simulink model "CLLLC_Plant_vLoad_V2"  (R2022a)
settings: Solver=FixedStepDiscrete  StartTime=0.0  StopTime=0.5  FixedStep=Step_Rate  RelTol=1e-3
model workspace (MAT data in the model file):
  CVI_INit = 0
  Fsw : Simulink.Signal (value not decoded)
  L_Lim = 0.6
  fnerr : Simulink.Signal (value not decoded)
  fsw : Simulink.Signal (value not decoded)
  swit : Simulink.Signal (value not decoded)
  tsw : Simulink.Signal (value not decoded)
values from neighbouring files (symbols this model uses):
  a0_cv_F = 0.01392699    [CLLLC_Plant_Parameters_vLoad_V2.m]
  a1_cv_F = -0.0060730    (= -0.006073)    [CLLLC_Plant_Parameters_vLoad_V2.m]
  a2_cv_F = 0.0    (= 0)    [CLLLC_Plant_Parameters_vLoad_V2.m]
  b1_cv_F = -1    [CLLLC_Plant_Parameters_vLoad_V2.m]
  b2_cv_F = 0.0    (= 0)    [CLLLC_Plant_Parameters_vLoad_V2.m]
  Cmd_Ref_Ctrl = round(Cmd_Ref * KVpri / VADC * ADCFS)    [CLLLC_Plant_Parameters_vLoad_V2.m]
  Control_Step_Rate = 50e-6    (= 5e-05)    [CLLLC_Plant_Parameters_vLoad_V2.m]
  Freq_Sw = 55.1e3    (= 55100)    [CLLLC_Plant_Parameters_vLoad_V2.m]
  KIout = 20e-3    (= 0.02)    [CLLLC_Plant_Parameters_vLoad_V2.m]
  KVpri = 0.0036102    [CLLLC_Plant_Parameters_vLoad_V2.m]
  KVsec = 0.00569815    [CLLLC_Plant_Parameters_vLoad_V2.m]
  Lm1 = Ln*LrP1    (= 8e-05)    [CLLLC_Plant_Parameters_vLoad_V2.m]
  n = 20.0/9.0    (= 2.22222222222)    [CLLLC_Plant_Parameters_vLoad_V2.m]
  R_series = 3    [CLLLC_Plant_Parameters_vLoad_V2.m]
  Reverse = 1    [CLLLC_Plant_Parameters_vLoad_V2.m]
  Step_Rate = 1e-7    (= 1e-07)    [CLLLC_Plant_Parameters_vLoad_V2.m]
  transformerCoupling = 0.999    [CLLLC_Plant_Parameters_vLoad_V2.m]
  Ts_Sw = floor(Fclk/Freq_Sw)    [CLLLC_Plant_Parameters_vLoad_V2.m]
libraries: fl_lib x36, nesl_utility x25, ee_lib x15, simulink x7, spsFirstOrderFilterLib x5, slpidlib x3, simulink_extras x3, eeGeneralControl x1
(part 3 of 3)

== system CLLLC_Plant_vLoad_V2/Loop Selection/Open Loop 1 ==
  note: 0 - SR Disable
      | 1 - SR Enable
  Constant : Constant  Value=0
  Mode Selection : Subsystem  Variant=on
  PWM_freq : Outport
  SR_En : Outport  Port=2
  wires:
  Constant/1 -> SR_En/1
  Mode Selection/1(PWM_Freq) -> PWM_freq/1

== system CLLLC_Plant_vLoad_V2/Loop Selection/Closed Loop/Mode Selection ==
  note: 1) Add Subsystem or Model blocks as valid variant choices.
      | 2) You cannot connect blocks at this level. At simulation, connectivity is automatically
      | determined, based on the active variant and port name matching.
  CC Mode : Subsystem  VariantControl=Charger_Mode == 0
  CV Mode Forward : Subsystem  VariantControl=Charger_Mode == 1
  CV Mode Reverse : Subsystem  VariantControl=Charger_Mode == 2
  PWM_Freq : Outport

== system CLLLC_Plant_vLoad_V2/Loop Selection/Closed Loop1/Mode Selection ==
  note: 1) Add Subsystem or Model blocks as valid variant choices.
      | 2) You cannot connect blocks at this level. At simulation, connectivity is automatically
      | determined, based on the active variant and port name matching.
  CC Mode : Subsystem  VariantControl=Charger_Mode == 0
  CV Mode Forward : Subsystem  VariantControl=Charger_Mode == 1
  CV Mode Reverse : Subsystem  VariantControl=Charger_Mode == 2
  PWM_freq : Outport

== system CLLLC_Plant_vLoad_V2/Loop Selection/Open Loop 1/Mode Selection ==
  note: 1) Add Subsystem or Model blocks as valid variant choices.
      | 2) You cannot connect blocks at this level. At simulation, connectivity is automatically
      | determined, based on the active variant and port name matching.
  CC Mode : Subsystem  VariantControl=Charger_Mode == 0
  CV Mode : Subsystem  VariantControl=Charger_Mode == 1
  PWM_Freq : Outport

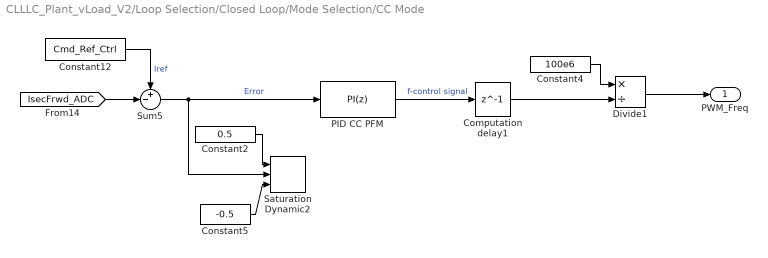
== system CLLLC_Plant_vLoad_V2/Loop Selection/Closed Loop/Mode Selection/CC Mode ==
  Computation delay1 : Delay  DelayLength=1  InitialCondition=200
  Constant12 : Constant  Value=Cmd_Ref_Ctrl
  Constant2 : Constant  Value=0.5
  Constant4 : Constant  Value=100e6
  Constant5 : Constant  Value=-0.5
  Divide1 : Product  Inputs=*/
  PID CC PFM : slpidlib/PID Controller  Controller=PI  Form=Parallel  TimeDomain=Discrete-time  UseExternalTs=off  SampleTime=Control_Step_Rate  IntegratorMethod=Forward Euler  FilterMethod=Forward Euler  ControllerParametersSource=internal  P=0.0661065319076132  I=416.251558932139  UseKiTs=off  D=-0.0462494978274742  N=100  UseFilter=off  TunerSelectOption=Transfer Function Based (PID Tuner App)  InitialConditionSource=internal  InitialConditionForIntegrator=200  InitialConditionForFilter=0  DifferentiatorICPrevScaledInput=0  ExternalReset=none  TrackingMode=off  Kt=1  LimitOutput=on  SatLimitsSource=internal  UpperSaturationLimit=750  LowerSaturationLimit=200  LinearizeAsGain=on  AntiWindupMode=back-calculation  Kb=1  POutMin=[]  POutMax=[]  IOutMin=[]  IOutMax=[]  DOutMin=[]  DOutMax=[]  NOutMin=[]  NOutMax=[]  SumOutMin=[]  SumOutMax=[]  SaturationOutMin=[]  SaturationOutMax=[]  PParamMin=[]  PParamMax=[]  IParamMin=[]  IParamMax=[]  DParamMin=[]  DParamMax=[]  NParamMin=[]  NParamMax=[]  KbParamMin=[]  KbParamMax=[]  KtParamMin=[]  KtParamMax=[]  KbOutMin=[]  KbOutMax=[]  KtOutMin=[]  KtOutMax=[]  IntegratorOutMin=[]  IntegratorOutMax=[]  FilterOutMin=[]  FilterOutMax=[]  SumI1OutMin=[]  SumI1OutMax=[]  SumI2OutMin=[]  SumI2OutMax=[]  SumI3OutMin=[]  SumI3OutMax=[]  SumI4OutMin=[]  SumI4OutMax=[]  SumDOutMin=[]  SumDOutMax=[]  DifferentiatorOutMin=[]  DifferentiatorOutMax=[]  FilterDiffOutCoefMin=[]  FilterDiffOutCoefMax=[]  ReciprocalOutMin=[]  ReciprocalOutMax=[]  SumDenOutMin=[]  SumDenOutMax=[]  SumNumOutMin=[]  SumNumOutMax=[]  DivideOutMin=[]  DivideOutMax=[]  UdiffTsProdOutMin=[]  UdiffTsProdOutMax=[]  NTsProdOutMin=[]  NTsProdOutMax=[]  UintegralTsProdOutMin=[]  UintegralTsProdOutMax=[]  UngainTsProdOutMin=[]  UngainTsProdOutMax=[]  IntegratorContinuousStateAttributes=''  IntegratorStateMustResolveToSignalObject=off  IntegratorRTWStateStorageClass=Auto  FilterContinuousStateAttributes=''  FilterStateMustResolveToSignalObject=off  FilterRTWStateStorageClass=Auto  ParallelPVariant=InternalParameters  IdealPVariant=Disabled  IVariant=InternalParameters  DVariant=Disabled  IntegratorVariant=Discrete  SatVariant=Enabled  AWVariant=BackCalculation  PCopyVariant=Disabled  TRVariant=Disabled  FdbkBlocksVariant=Forward  IdealPFdbkVariant=Disabled  SatFdbkVariant=Disabled  DerivativeFilterVariant=Disabled  NVariant=Disabled  NCopyVariant=Disabled_SignalSpec  FilterICVariant=Disabled  IntegratorICVariant=InternalICs  ExternalResetVariant=Disabled  TRSumVariant=Passthrough  SumFdbkVariant=Disabled  SumVariant=Sum_PI  TsampFilterVariant=InternalTs  TsampNgainVariant=Passthrough  TsampIntegralVariant=Passthrough  ExternalSaturationOutDataTypeStr=Inherit: Same as second input  aMode=0
  Saturation Dynamic2 : simulink/Discontinuities/Saturation Dynamic  OutMin=[]  OutMax=[]  OutDataTypeStr=Inherit: Same as second input  OutDataType=fixdt(1, 16)  OutScaling=2^-10  DoSatur=off
  Sum5 : Sum  Inputs=+-|
  PWM_Freq : Outport
  wires:
  PID CC PFM/1 -> Computation delay1/1  "f-control signal"
  Constant2/1 -> Saturation Dynamic2/1
  Sum5/1 -> Saturation Dynamic2/2, PID CC PFM/1  "Error"
  Constant5/1 -> Saturation Dynamic2/3
  [IsecFrwd_ADC] -> Sum5/2
  Constant12/1 -> Sum5/1  "Iref"
  Constant4/1 -> Divide1/1
  Computation delay1/1 -> Divide1/2
  Divide1/1 -> PWM_Freq/1

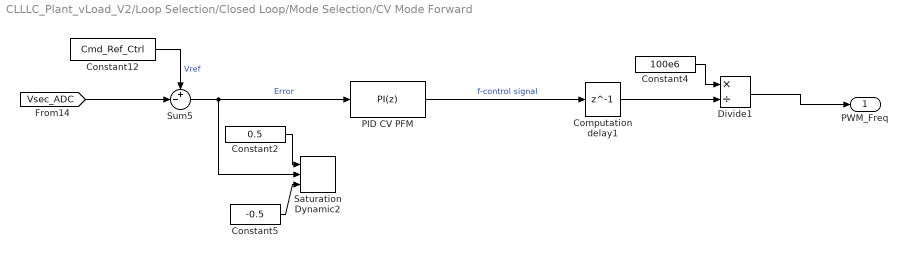
== system CLLLC_Plant_vLoad_V2/Loop Selection/Closed Loop/Mode Selection/CV Mode Forward ==
  Computation delay1 : Delay  DelayLength=1  InitialCondition=200
  Constant12 : Constant  Value=Cmd_Ref_Ctrl
  Constant2 : Constant  Value=0.5
  Constant4 : Constant  Value=100e6
  Constant5 : Constant  Value=-0.5
  Divide1 : Product  Inputs=*/
  PID CV PFM : slpidlib/PID Controller  Controller=PI  Form=Parallel  TimeDomain=Discrete-time  UseExternalTs=off  SampleTime=Control_Step_Rate  IntegratorMethod=Forward Euler  FilterMethod=Forward Euler  ControllerParametersSource=internal  P=0.068496  I=349.9686  UseKiTs=off  D=-0.0462494978274742  N=100  UseFilter=off  TunerSelectOption=Transfer Function Based (PID Tuner App)  InitialConditionSource=internal  InitialConditionForIntegrator=200  InitialConditionForFilter=0  DifferentiatorICPrevScaledInput=0  ExternalReset=none  TrackingMode=off  Kt=1  LimitOutput=on  SatLimitsSource=internal  UpperSaturationLimit=750  LowerSaturationLimit=200  LinearizeAsGain=on  AntiWindupMode=back-calculation  Kb=1  POutMin=[]  POutMax=[]  IOutMin=[]  IOutMax=[]  DOutMin=[]  DOutMax=[]  NOutMin=[]  NOutMax=[]  SumOutMin=[]  SumOutMax=[]  SaturationOutMin=[]  SaturationOutMax=[]  PParamMin=[]  PParamMax=[]  IParamMin=[]  IParamMax=[]  DParamMin=[]  DParamMax=[]  NParamMin=[]  NParamMax=[]  KbParamMin=[]  KbParamMax=[]  KtParamMin=[]  KtParamMax=[]  KbOutMin=[]  KbOutMax=[]  KtOutMin=[]  KtOutMax=[]  IntegratorOutMin=[]  IntegratorOutMax=[]  FilterOutMin=[]  FilterOutMax=[]  SumI1OutMin=[]  SumI1OutMax=[]  SumI2OutMin=[]  SumI2OutMax=[]  SumI3OutMin=[]  SumI3OutMax=[]  SumI4OutMin=[]  SumI4OutMax=[]  SumDOutMin=[]  SumDOutMax=[]  DifferentiatorOutMin=[]  DifferentiatorOutMax=[]  FilterDiffOutCoefMin=[]  FilterDiffOutCoefMax=[]  ReciprocalOutMin=[]  ReciprocalOutMax=[]  SumDenOutMin=[]  SumDenOutMax=[]  SumNumOutMin=[]  SumNumOutMax=[]  DivideOutMin=[]  DivideOutMax=[]  UdiffTsProdOutMin=[]  UdiffTsProdOutMax=[]  NTsProdOutMin=[]  NTsProdOutMax=[]  UintegralTsProdOutMin=[]  UintegralTsProdOutMax=[]  UngainTsProdOutMin=[]  UngainTsProdOutMax=[]  IntegratorContinuousStateAttributes=''  IntegratorStateMustResolveToSignalObject=off  IntegratorRTWStateStorageClass=Auto  FilterContinuousStateAttributes=''  FilterStateMustResolveToSignalObject=off  FilterRTWStateStorageClass=Auto  ParallelPVariant=InternalParameters  IdealPVariant=Disabled  IVariant=InternalParameters  DVariant=Disabled  IntegratorVariant=Discrete  SatVariant=Enabled  AWVariant=BackCalculation  PCopyVariant=Disabled  TRVariant=Disabled  FdbkBlocksVariant=Forward  IdealPFdbkVariant=Disabled  SatFdbkVariant=Disabled  DerivativeFilterVariant=Disabled  NVariant=Disabled  NCopyVariant=Disabled_SignalSpec  FilterICVariant=Disabled  IntegratorICVariant=InternalICs  ExternalResetVariant=Disabled  TRSumVariant=Passthrough  SumFdbkVariant=Disabled  SumVariant=Sum_PI  TsampFilterVariant=InternalTs  TsampNgainVariant=Passthrough  TsampIntegralVariant=Passthrough  ExternalSaturationOutDataTypeStr=Inherit: Same as second input  aMode=0
  Saturation Dynamic2 : simulink/Discontinuities/Saturation Dynamic  OutMin=[]  OutMax=[]  OutDataTypeStr=Inherit: Same as second input  OutDataType=fixdt(1, 16)  OutScaling=2^-10  DoSatur=off
  Sum5 : Sum  Inputs=+-|
  PWM_Freq : Outport
  wires:
  Constant2/1 -> Saturation Dynamic2/1
  Sum5/1 -> Saturation Dynamic2/2, PID CV PFM/1  "Error"
  Constant5/1 -> Saturation Dynamic2/3
  PID CV PFM/1 -> Computation delay1/1  "f-control signal"
  Constant12/1 -> Sum5/1  "Vref"
  Constant4/1 -> Divide1/1
  Divide1/1 -> PWM_Freq/1
  [Vsec_ADC] -> Sum5/2
  Computation delay1/1 -> Divide1/2

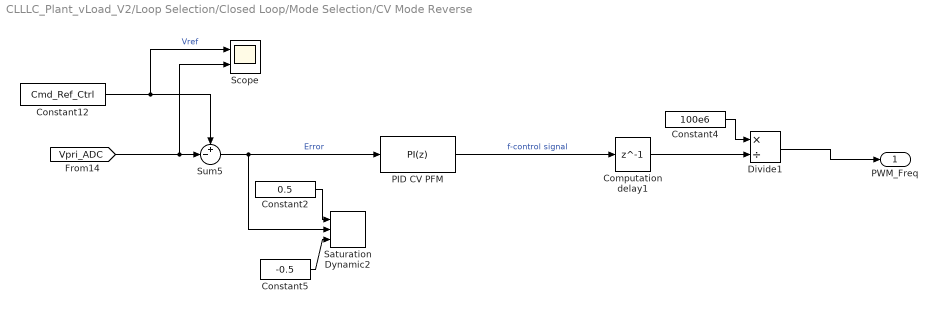
== system CLLLC_Plant_vLoad_V2/Loop Selection/Closed Loop/Mode Selection/CV Mode Reverse ==
  Computation delay1 : Delay  DelayLength=1  InitialCondition=200
  Constant12 : Constant  Value=Cmd_Ref_Ctrl
  Constant2 : Constant  Value=0.5
  Constant4 : Constant  Value=100e6
  Constant5 : Constant  Value=-0.5
  Divide1 : Product  Inputs=*/
  PID CV PFM : slpidlib/PID Controller  Controller=PI  Form=Parallel  TimeDomain=Discrete-time  UseExternalTs=off  SampleTime=Control_Step_Rate  IntegratorMethod=Forward Euler  FilterMethod=Forward Euler  ControllerParametersSource=internal  P=0.170506780572651  I=9.31712886047831  UseKiTs=off  D=-0.0462494978274742  N=100  UseFilter=off  TunerSelectOption=Transfer Function Based (PID Tuner App)  InitialConditionSource=internal  InitialConditionForIntegrator=361  InitialConditionForFilter=0  DifferentiatorICPrevScaledInput=0  ExternalReset=none  TrackingMode=off  Kt=1  LimitOutput=on  SatLimitsSource=internal  UpperSaturationLimit=750  LowerSaturationLimit=200  LinearizeAsGain=on  AntiWindupMode=back-calculation  Kb=1  POutMin=[]  POutMax=[]  IOutMin=[]  IOutMax=[]  DOutMin=[]  DOutMax=[]  NOutMin=[]  NOutMax=[]  SumOutMin=[]  SumOutMax=[]  SaturationOutMin=[]  SaturationOutMax=[]  PParamMin=[]  PParamMax=[]  IParamMin=[]  IParamMax=[]  DParamMin=[]  DParamMax=[]  NParamMin=[]  NParamMax=[]  KbParamMin=[]  KbParamMax=[]  KtParamMin=[]  KtParamMax=[]  KbOutMin=[]  KbOutMax=[]  KtOutMin=[]  KtOutMax=[]  IntegratorOutMin=[]  IntegratorOutMax=[]  FilterOutMin=[]  FilterOutMax=[]  SumI1OutMin=[]  SumI1OutMax=[]  SumI2OutMin=[]  SumI2OutMax=[]  SumI3OutMin=[]  SumI3OutMax=[]  SumI4OutMin=[]  SumI4OutMax=[]  SumDOutMin=[]  SumDOutMax=[]  DifferentiatorOutMin=[]  DifferentiatorOutMax=[]  FilterDiffOutCoefMin=[]  FilterDiffOutCoefMax=[]  ReciprocalOutMin=[]  ReciprocalOutMax=[]  SumDenOutMin=[]  SumDenOutMax=[]  SumNumOutMin=[]  SumNumOutMax=[]  DivideOutMin=[]  DivideOutMax=[]  UdiffTsProdOutMin=[]  UdiffTsProdOutMax=[]  NTsProdOutMin=[]  NTsProdOutMax=[]  UintegralTsProdOutMin=[]  UintegralTsProdOutMax=[]  UngainTsProdOutMin=[]  UngainTsProdOutMax=[]  IntegratorContinuousStateAttributes=''  IntegratorStateMustResolveToSignalObject=off  IntegratorRTWStateStorageClass=Auto  FilterContinuousStateAttributes=''  FilterStateMustResolveToSignalObject=off  FilterRTWStateStorageClass=Auto  ParallelPVariant=InternalParameters  IdealPVariant=Disabled  IVariant=InternalParameters  DVariant=Disabled  IntegratorVariant=Discrete  SatVariant=Enabled  AWVariant=BackCalculation  PCopyVariant=Disabled  TRVariant=Disabled  FdbkBlocksVariant=Forward  IdealPFdbkVariant=Disabled  SatFdbkVariant=Disabled  DerivativeFilterVariant=Disabled  NVariant=Disabled  NCopyVariant=Disabled_SignalSpec  FilterICVariant=Disabled  IntegratorICVariant=InternalICs  ExternalResetVariant=Disabled  TRSumVariant=Passthrough  SumFdbkVariant=Disabled  SumVariant=Sum_PI  TsampFilterVariant=InternalTs  TsampNgainVariant=Passthrough  TsampIntegralVariant=Passthrough  ExternalSaturationOutDataTypeStr=Inherit: Same as second input  aMode=0
  Saturation Dynamic2 : simulink/Discontinuities/Saturation Dynamic  OutMin=[]  OutMax=[]  OutDataTypeStr=Inherit: Same as second input  OutDataType=fixdt(1, 16)  OutScaling=2^-10  DoSatur=off
  Scope : Scope  NumInputPorts=2
  Sum5 : Sum  Inputs=+-|
  PWM_Freq : Outport
  wires:
  Constant2/1 -> Saturation Dynamic2/1
  Sum5/1 -> Saturation Dynamic2/2, PID CV PFM/1  "Error"
  Constant5/1 -> Saturation Dynamic2/3
  PID CV PFM/1 -> Computation delay1/1  "f-control signal"
  Constant12/1 -> Scope/1, Sum5/1  "Vref"
  Constant4/1 -> Divide1/1
  Divide1/1 -> PWM_Freq/1
  [Vpri_ADC] -> Scope/2, Sum5/2
  Computation delay1/1 -> Divide1/2

== system CLLLC_Plant_vLoad_V2/Loop Selection/Closed Loop1/Mode Selection/CC Mode ==
  Constant12 : Constant  Value=Cmd_Ref_Ctrl
  Subsystem : Subsystem
  PWM_freq : Outport
  wires:
  [IsecFrwd_ADC] -> Subsystem/2(In2)
  [Control_step_timer] -> Subsystem/Trigger
  Subsystem/1(PWM_freq) -> PWM_freq/1
  Constant12/1 -> Subsystem/1(Iref)  "Iref"

== system CLLLC_Plant_vLoad_V2/Loop Selection/Closed Loop1/Mode Selection/CV Mode Forward ==
  Constant12 : Constant  Value=Cmd_Ref_Ctrl
  Subsystem : Subsystem
  PWM_freq : Outport
  wires:
  Constant12/1 -> Subsystem/1(Vref)  "Vref"
  [Vsec_ADC] -> Subsystem/2(In2)
  Subsystem/1(Out1) -> PWM_freq/1
  [Control_step_timer] -> Subsystem/Trigger

== system CLLLC_Plant_vLoad_V2/Loop Selection/Closed Loop1/Mode Selection/CV Mode Reverse ==
  Constant12 : Constant  Value=Cmd_Ref_Ctrl
  Subsystem : Subsystem
  PWM_freq : Outport
  wires:
  Constant12/1 -> Subsystem/1(Vref)  "Vref"
  [Vpri_ADC] -> Subsystem/2(In2)
  Subsystem/1(Out1) -> PWM_freq/1
  [Control_step_timer] -> Subsystem/Trigger

== system CLLLC_Plant_vLoad_V2/Loop Selection/Open Loop 1/Mode Selection/CC Mode ==
  Constant4 : Constant  Value=100e6
  Constant5 : Constant  Value=Ts_Sw
  Divide1 : Product  Inputs=*/
  PWM_Freq : Outport
  wires:
  Constant5/1 -> Divide1/2  "f-control signal"
  Constant4/1 -> Divide1/1
  Divide1/1 -> PWM_Freq/1

== system CLLLC_Plant_vLoad_V2/Loop Selection/Open Loop 1/Mode Selection/CV Mode ==
  note: f-control signal
  Constant4 : Constant  Value=100e6
  Constant5 : Constant  Value=Ts_Sw
  Divide1 : Product  Inputs=*/
  PWM_Freq : Outport
  wires:
  Constant5/1 -> Divide1/2
  Constant4/1 -> Divide1/1
  Divide1/1 -> PWM_Freq/1

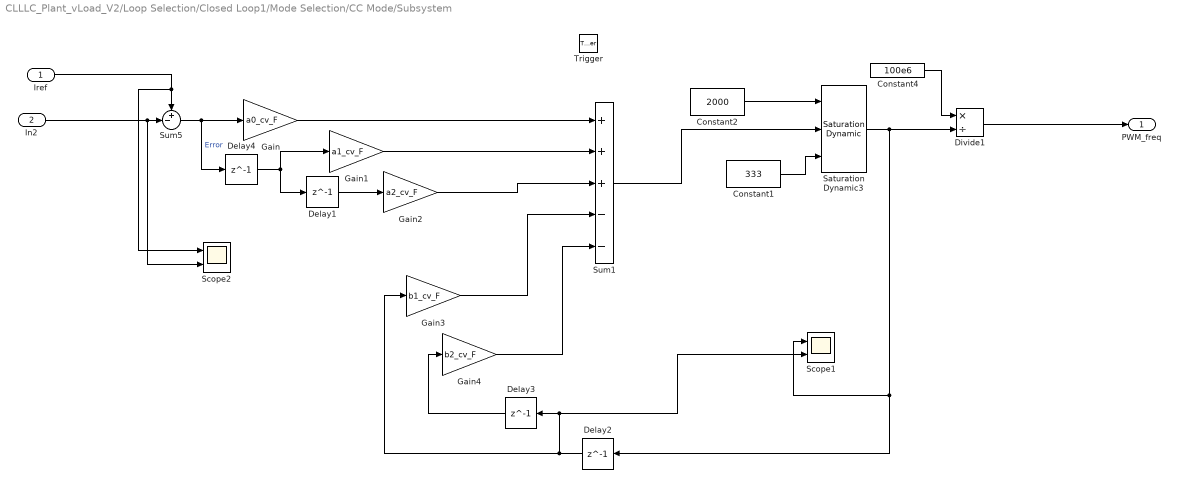
== system CLLLC_Plant_vLoad_V2/Loop Selection/Closed Loop1/Mode Selection/CC Mode/Subsystem ==
  Iref : Inport
  In2 : Inport  Port=2
  Trigger : TriggerPort  VariantControl=Variant  PortDimensions=1
  Constant1 : Constant  Value=333  OutDataTypeStr=single
  Constant2 : Constant  Value=2000  OutDataTypeStr=single
  Constant4 : Constant  Value=100e6
  Delay1 : Delay  DelayLength=1  InitialCondition=0
  Delay2 : Delay  DelayLength=1  InitialCondition=125
  Delay3 : Delay  DelayLength=1  InitialCondition=125
  Delay4 : Delay  DelayLength=1  InitialCondition=0
  Divide1 : Product  Inputs=*/
  Gain : Gain  Gain=a0_cv_F
  Gain1 : Gain  Gain=a1_cv_F
  Gain2 : Gain  Gain=a2_cv_F
  Gain3 : Gain  Gain=b1_cv_F
  Gain4 : Gain  Gain=b2_cv_F
  Saturation Dynamic3 : simulink/Discontinuities/Saturation Dynamic  OutMin=[]  OutMax=[]  OutDataTypeStr=Inherit: Same as second input  OutDataType=fixdt(1, 16)  OutScaling=2^-10  DoSatur=off
  Scope1 : Scope  NumInputPorts=2
  Scope2 : Scope  NumInputPorts=2
  Sum1 : Sum  Inputs=+++--
  Sum5 : Sum  Inputs=+-|
  PWM_freq : Outport
  wires:
  Saturation Dynamic3/1 -> Delay2/1, Scope1/1, Divide1/2
  Constant1/1 -> Saturation Dynamic3/3
  Sum5/1 -> Gain/1, Delay4/1  "Error"
  Gain3/1 -> Sum1/4
  Constant2/1 -> Saturation Dynamic3/1
  Delay1/1 -> Gain2/1
  Gain1/1 -> Sum1/2
  Delay4/1 -> Delay1/1, Gain1/1
  Sum1/1 -> Saturation Dynamic3/2
  Delay3/1 -> Gain4/1
  Delay2/1 -> Gain3/1, Scope1/2, Delay3/1
  Divide1/1 -> PWM_freq/1
  Gain/1 -> Sum1/1
  Iref/1 -> Sum5/1, Scope2/1
  Gain4/1 -> Sum1/5
  Gain2/1 -> Sum1/3
  Constant4/1 -> Divide1/1
  In2/1 -> Scope2/2, Sum5/2

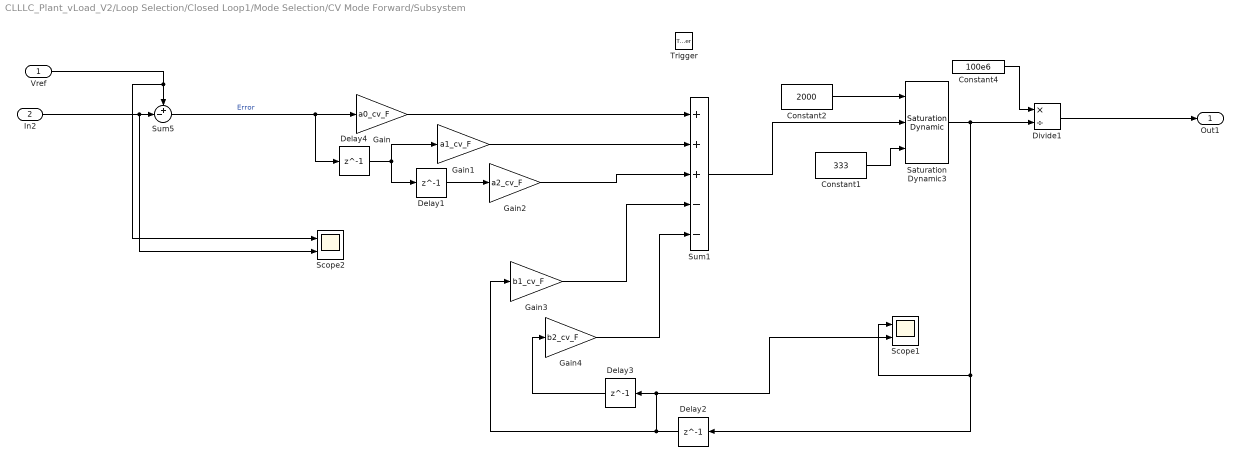
== system CLLLC_Plant_vLoad_V2/Loop Selection/Closed Loop1/Mode Selection/CV Mode Forward/Subsystem ==
  Vref : Inport
  In2 : Inport  Port=2
  Trigger : TriggerPort  VariantControl=Variant  PortDimensions=1
  Constant1 : Constant  Value=333  OutDataTypeStr=single
  Constant2 : Constant  Value=2000  OutDataTypeStr=single
  Constant4 : Constant  Value=100e6
  Delay1 : Delay  DelayLength=1  InitialCondition=0
  Delay2 : Delay  DelayLength=1  InitialCondition=125
  Delay3 : Delay  DelayLength=1  InitialCondition=125
  Delay4 : Delay  DelayLength=1  InitialCondition=0
  Divide1 : Product  Inputs=*/
  Gain : Gain  Gain=a0_cv_F
  Gain1 : Gain  Gain=a1_cv_F
  Gain2 : Gain  Gain=a2_cv_F
  Gain3 : Gain  Gain=b1_cv_F
  Gain4 : Gain  Gain=b2_cv_F
  Saturation Dynamic3 : simulink/Discontinuities/Saturation Dynamic  OutMin=[]  OutMax=[]  OutDataTypeStr=Inherit: Same as second input  OutDataType=fixdt(1, 16)  OutScaling=2^-10  DoSatur=off
  Scope1 : Scope  NumInputPorts=2
  Scope2 : Scope  NumInputPorts=2
  Sum1 : Sum  Inputs=+++--
  Sum5 : Sum  Inputs=+-|
  Out1 : Outport
  wires:
  Saturation Dynamic3/1 -> Delay2/1, Scope1/1, Divide1/2
  Constant1/1 -> Saturation Dynamic3/3
  Sum5/1 -> Gain/1, Delay4/1  "Error"
  Gain3/1 -> Sum1/4
  Constant2/1 -> Saturation Dynamic3/1
  Delay1/1 -> Gain2/1
  Gain1/1 -> Sum1/2
  Delay4/1 -> Delay1/1, Gain1/1
  Sum1/1 -> Saturation Dynamic3/2
  Delay3/1 -> Gain4/1
  Delay2/1 -> Gain3/1, Scope1/2, Delay3/1
  Divide1/1 -> Out1/1
  Gain/1 -> Sum1/1
  Vref/1 -> Sum5/1, Scope2/1
  Gain4/1 -> Sum1/5
  Gain2/1 -> Sum1/3
  Constant4/1 -> Divide1/1
  In2/1 -> Scope2/2, Sum5/2

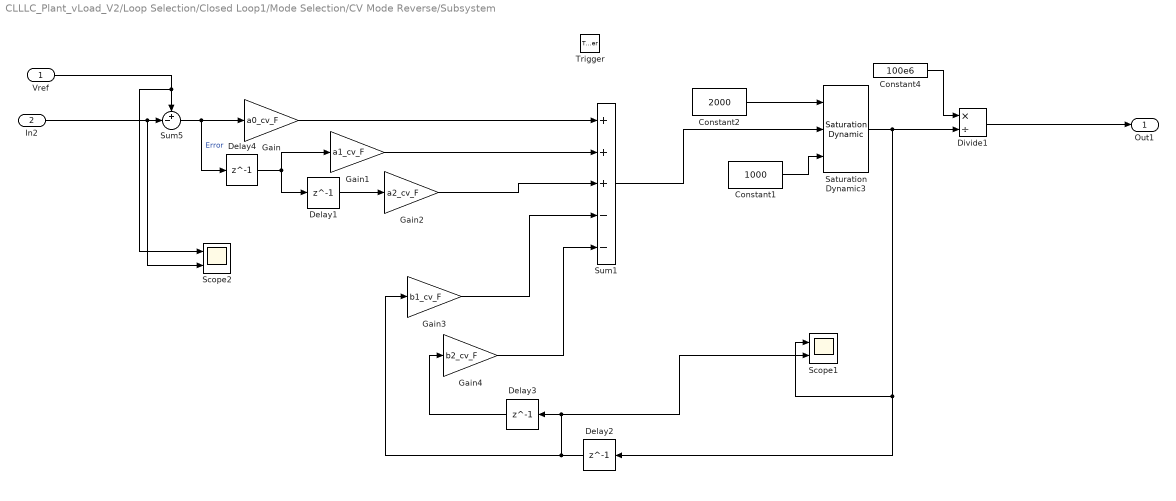
== system CLLLC_Plant_vLoad_V2/Loop Selection/Closed Loop1/Mode Selection/CV Mode Reverse/Subsystem ==
  Vref : Inport
  In2 : Inport  Port=2
  Trigger : TriggerPort  VariantControl=Variant  PortDimensions=1
  Constant1 : Constant  Value=1000  OutDataTypeStr=single
  Constant2 : Constant  Value=2000  OutDataTypeStr=single
  Constant4 : Constant  Value=100e6
  Delay1 : Delay  DelayLength=1  InitialCondition=0
  Delay2 : Delay  DelayLength=1  InitialCondition=346
  Delay3 : Delay  DelayLength=1  InitialCondition=346
  Delay4 : Delay  DelayLength=1  InitialCondition=0
  Divide1 : Product  Inputs=*/
  Gain : Gain  Gain=a0_cv_F
  Gain1 : Gain  Gain=a1_cv_F
  Gain2 : Gain  Gain=a2_cv_F
  Gain3 : Gain  Gain=b1_cv_F
  Gain4 : Gain  Gain=b2_cv_F
  Saturation Dynamic3 : simulink/Discontinuities/Saturation Dynamic  OutMin=[]  OutMax=[]  OutDataTypeStr=Inherit: Same as second input  OutDataType=fixdt(1, 16)  OutScaling=2^-10  DoSatur=off
  Scope1 : Scope  NumInputPorts=2
  Scope2 : Scope  NumInputPorts=2
  Sum1 : Sum  Inputs=+++--
  Sum5 : Sum  Inputs=+-|
  Out1 : Outport
  wires:
  Saturation Dynamic3/1 -> Delay2/1, Scope1/1, Divide1/2
  Constant1/1 -> Saturation Dynamic3/3
  Sum5/1 -> Gain/1, Delay4/1  "Error"
  Gain3/1 -> Sum1/4
  Constant2/1 -> Saturation Dynamic3/1
  Delay1/1 -> Gain2/1
  Gain1/1 -> Sum1/2
  Delay4/1 -> Delay1/1, Gain1/1
  Sum1/1 -> Saturation Dynamic3/2
  Delay3/1 -> Gain4/1
  Delay2/1 -> Gain3/1, Scope1/2, Delay3/1
  Divide1/1 -> Out1/1
  Gain/1 -> Sum1/1
  Vref/1 -> Sum5/1, Scope2/1
  Gain4/1 -> Sum1/5
  Gain2/1 -> Sum1/3
  Constant4/1 -> Divide1/1
  In2/1 -> Scope2/2, Sum5/2

== matlab function CLLLC_Plant_vLoad_V2/Loop Selection/Open Loop/Open Loop Soft Start ==
  settings: updateMethod=DISCRETE
  data: Step_Rate parameter; PWM_Freq output; SR_EN output; Freq_Sw parameter
function [PWM_Freq, SR_EN] = OpenLoopSS(Step_Rate, Freq_Sw)
 
persistent PWM_Freq_Start
if isempty(PWM_Freq_Start) %Init
    PWM_Freq_Start = 200e3;
end
 
persistent PWM_Freq_Curr1
if isempty(PWM_Freq_Curr1) %Init
    PWM_Freq_Curr1 = PWM_Freq_Start;
end
 
persistent SS_Flag1
if isempty(SS_Flag1) %Init
    SS_Flag1 = 0;
end
 
Freq_Step = (PWM_Freq_Start - Freq_Sw) / (0.0001/Step_Rate);
 
if SS_Flag1 == 0
    if PWM_Freq_Curr1 <= Freq_Sw 
        SS_Flag1 = 1;
    else
        PWM_Freq_Curr1 = PWM_Freq_Curr1 - Freq_Step;
    end
else
    PWM_Freq_Curr1 = Freq_Sw;
end
 
PWM_Freq = PWM_Freq_Curr1;
 
if SS_Flag1 == 1 
    SR_EN = 0;
else
    SR_EN = 0;
end
 
end

== matlab function CLLLC_Plant_vLoad_V2/PWM Generator  CLLLC ==
  settings: updateMethod=DISCRETE
  data: PWM_Freq input; SR_En input; Step_Rate parameter; Reverse parameter; PWMPA output; PWMPB output; PWMSA output; PWMSB output; PRD output
function [PWMPA, PWMPB, PWMSA, PWMSB, PRD]   = PWM_Generator(PWM_Freq, SR_En, Step_Rate, Reverse)
 
persistent Period_Act
if isempty(Period_Act) %Init
    Period_Act = 0;
end
 
persistent Period_Count
if isempty(Period_Count) %Init
    Period_Count = 0;
end
 
persistent PWM1A_Stat 
if isempty(PWM1A_Stat) %Init
    PWM1A_Stat = 0;
end
 
persistent PWM1B_Stat 
if isempty(PWM1B_Stat) %Init
    PWM1B_Stat = 0;
end
 
persistent PWM2A_Stat 
if isempty(PWM2A_Stat) %Init
    PWM2A_Stat = 0;
end
 
persistent PWM2B_Stat 
if isempty(PWM2B_Stat) %Init
    PWM2B_Stat = 0;
end
 
persistent PWM1A_H 
if isempty(PWM1A_H) %Init
    PWM1A_H = 0;
end
 
persistent PWM1A_L 
if isempty(PWM1A_L) %Init
    PWM1A_L = 0;
end
 
persistent PWM1B_H 
if isempty(PWM1B_H) %Init
    PWM1B_H = 0;
end
 
persistent PWM1B_L 
if isempty(PWM1B_L) %Init
    PWM1B_L = 0;
end
 
persistent PWM2A_H 
if isempty(PWM2A_H) %Init
    PWM2A_H = 0;
end
 
persistent PWM2A_L 
if isempty(PWM2A_L) %Init
    PWM2A_L = 0;
end
 
persistent PWM2B_H 
if isempty(PWM2B_H) %Init
    PWM2B_H = 0;
end
 
persistent PWM2B_L 
if isempty(PWM2B_L) %Init
    PWM2B_L = 0;
end
 
Pri_Dead_Time = 0.25e-6 / Step_Rate;
Sec_Dead_Time = 0.5e-6 / Step_Rate;
 
Pri_DTime_Half_Count = Pri_Dead_Time / 2;
Sec_DTime_Half_Count = Sec_Dead_Time / 2;
 
if PWM_Freq <= 0
    PWM_Freq = 240000;
end
    
Period_Cmd = (1/PWM_Freq) / Step_Rate;
 
if Period_Count >= Period_Act
    Period_Count = 0;
        
    Period_Act = Period_Cmd;
        
    % Update Duty Count
    Duty_50 = Period_Cmd / 2;
    
    %Base Frequecny PWM With 50% Duty
    PWM1A_H = Pri_DTime_Half_Count;
    PWM1A_L = Duty_50 - Pri_DTime_Half_Count;      % -1 to Avoid Overflow
    
    PWM1B_H = Duty_50 + Pri_DTime_Half_Count;
    PWM1B_L = Period_Cmd - Pri_DTime_Half_Count;
    
    %With Phase Shift
    PWM2A_H = Sec_DTime_Half_Count;
    PWM2A_L = Duty_50 - Sec_DTime_Half_Count;      % -1 to Avoid Overflow
    
    PWM2B_H = Duty_50 + Sec_DTime_Half_Count;
    PWM2B_L = Period_Cmd - Sec_DTime_Half_Count;    
else
     Period_Count = Period_Count + 1; 
end
 
if Period_Count > PWM1A_L 
    PWM1A_Stat = 0;
elseif Period_Count > PWM1A_H       
    PWM1A_Stat = 1;
end
 
if Period_Count > PWM1B_L 
    PWM1B_Stat = 0;
elseif Period_Count > PWM1B_H         
    PWM1B_Stat = 1;
end
 
if Period_Count > PWM2A_L 
    PWM2A_Stat = 0;
elseif Period_Count > PWM2A_H       
    PWM2A_Stat = 1;
end
 
if Period_Count > PWM2B_L 
    PWM2B_Stat = 0;
elseif Period_Count > PWM2B_H         
    PWM2B_Stat = 1;
end
 
PWM_EN = 1;
 
%LLC Outputs
if PWM_EN == 1    
    if Reverse == 0        
        PWMPA = PWM1A_Stat;
        PWMPB = PWM1B_Stat;
 
        if SR_En == 1        
            PWMSA = PWM2A_Stat;
            PWMSB = PWM2B_Stat;
        else        
            PWMSA = 0;
            PWMSB = 0;
        end
    else        
        PWMSA = PWM1A_Stat;
        PWMSB = PWM1B_Stat;
 
        if SR_En == 1        
            PWMPA = PWM2A_Stat;
            PWMPB = PWM2B_Stat;
        else        
            PWMPA = 0;
            PWMPB = 0;
        end
    end
else
    PWMPA = 0;
    PWMPB = 0;
    PWMSA = 0;
    PWMSB = 0;
end

if Period_Count >= Period_Act
    PRD = 1;
else
    PRD = 0;
end
 
end

== matlab function CLLLC_Plant_vLoad_V2/SR Control Sec H ==
  settings: updateMethod=DISCRETE
  data: ITx input; PWM_Trig input; PWM_SR output; Step_Rate parameter
function PWM_SR    = SR_Control(ITx, PWM_Trig, Step_Rate)
 %Constant defines
 
persistent SR_Signal
if isempty(SR_Signal) %Init
    SR_Signal = 0;
end

persistent SR_State
if isempty(SR_State) %Init
    SR_State = 0;
end

persistent PWM_TRIG_State
if isempty(PWM_TRIG_State) %Init
    PWM_TRIG_State = 0;
end

persistent SR_Trig_Count
if isempty(SR_Trig_Count) %Init
    SR_Trig_Count = 0;
end

%SR Trigger Limits - High Side
SR_H_LIM = 8.0;
SR_L_LIM = 5.0;    
SR_H_Trig_Delay = 0.120e-6 / Step_Rate;

if PWM_TRIG_State == 0 %Init
    if PWM_Trig == 0
        PWM_TRIG_State = 1;
    end
elseif PWM_TRIG_State == 1 % Low State Waiting for Raising Edge    
    if PWM_Trig == 1
        PWM_TRIG_State = 2;
    end
elseif PWM_TRIG_State == 2 % Raising Edge Detected 
    PWM_TRIG_State = 3;
elseif PWM_TRIG_State == 3 % @ High State - Wait for Low State 
     if PWM_Trig == 0
        PWM_TRIG_State = 1;
    end
end

if SR_State == 0
    if ITx > SR_H_LIM
        SR_Trig_Count = SR_Trig_Count + 1;
        if SR_Trig_Count > SR_H_Trig_Delay
            SR_State = 1;
            SR_Signal = 1;   
            SR_Trig_Count = 0;
        end
    else
        SR_Trig_Count = 0;        
    end
elseif  SR_State == 1
    if ITx < SR_L_LIM
       SR_Signal = 0;   
       SR_State = 2;
    end
elseif  SR_State == 2
    if PWM_TRIG_State == 2 
        %if raising edge Detected
        SR_State = 0;
    end    
end     

if SR_Signal == 1
    PWM_SR = 1;
else
    PWM_SR = 0;    
end    

end

== matlab function CLLLC_Plant_vLoad_V2/SR Control Sec L ==
  settings: updateMethod=DISCRETE
  data: ITx input; PWM_Trig input; PWM_SR output; Step_Rate parameter
function PWM_SR    = SR_Control(ITx, PWM_Trig, Step_Rate)
 %Constant defines
 
persistent SR_Signal
if isempty(SR_Signal) %Init
    SR_Signal = 0;
end

persistent SR_State
if isempty(SR_State) %Init
    SR_State = 0;
end

persistent PWM_TRIG_State
if isempty(PWM_TRIG_State) %Init
    PWM_TRIG_State = 0;
end

persistent SR_Trig_Count
if isempty(SR_Trig_Count) %Init
    SR_Trig_Count = 0;
end

%SR Trigger Limits - High Side
SR_H_LIM = -8.0;
SR_L_LIM = -5.0;    
SR_H_Trig_Delay = 0.120e-6 / Step_Rate;

if PWM_TRIG_State == 0 %Init
    if PWM_Trig == 0
        PWM_TRIG_State = 1;
    end
elseif PWM_TRIG_State == 1 % Low State Waiting for Raising Edge    
    if PWM_Trig == 1
        PWM_TRIG_State = 2;
    end
elseif PWM_TRIG_State == 2 % Raising Edge Detected 
    PWM_TRIG_State = 3;
elseif PWM_TRIG_State == 3 % @ High State - Wait for Low State 
     if PWM_Trig == 0
        PWM_TRIG_State = 1;
    end
end

if SR_State == 0
    if ITx < SR_H_LIM
        SR_Trig_Count = SR_Trig_Count + 1;
        if SR_Trig_Count > SR_H_Trig_Delay
            SR_State = 1;
            SR_Signal = 1;   
            SR_Trig_Count = 0;
        end
    else
        SR_Trig_Count = 0;        
    end
elseif  SR_State == 1
    if ITx > SR_L_LIM
       SR_Signal = 0;   
       SR_State = 2;
    end
elseif  SR_State == 2
    if PWM_TRIG_State == 2 
        %if raising edge Detected
        SR_State = 0;
    end    
end     

if SR_Signal == 1
    PWM_SR = 1;
else
    PWM_SR = 0;    
end    

end

== matlab function CLLLC_Plant_vLoad_V2/SR Control Pri H ==
  settings: updateMethod=DISCRETE
  data: ITx input; PWM_Trig input; PWM_SR output; Step_Rate parameter
function PWM_SR    = SR_Control(ITx, PWM_Trig, Step_Rate)
 %Constant defines
 
persistent SR_Signal
if isempty(SR_Signal) %Init
    SR_Signal = 0;
end

persistent SR_State
if isempty(SR_State) %Init
    SR_State = 0;
end

persistent PWM_TRIG_State
if isempty(PWM_TRIG_State) %Init
    PWM_TRIG_State = 0;
end

persistent SR_Trig_Count
if isempty(SR_Trig_Count) %Init
    SR_Trig_Count = 0;
end

%SR Trigger Limits - High Side
SR_H_LIM = 8.0;
SR_L_LIM = 5.0;    
SR_H_Trig_Delay = 0.120e-6 / Step_Rate;

if PWM_TRIG_State == 0 %Init
    if PWM_Trig == 0
        PWM_TRIG_State = 1;
    end
elseif PWM_TRIG_State == 1 % Low State Waiting for Raising Edge    
    if PWM_Trig == 1
        PWM_TRIG_State = 2;
    end
elseif PWM_TRIG_State == 2 % Raising Edge Detected 
    PWM_TRIG_State = 3;
elseif PWM_TRIG_State == 3 % @ High State - Wait for Low State 
     if PWM_Trig == 0
        PWM_TRIG_State = 1;
    end
end

if SR_State == 0
    if ITx > SR_H_LIM
        SR_Trig_Count = SR_Trig_Count + 1;
        if SR_Trig_Count > SR_H_Trig_Delay
            SR_State = 1;
            SR_Signal = 1;   
            SR_Trig_Count = 0;
        end
    else
        SR_Trig_Count = 0;        
    end
elseif  SR_State == 1
    if ITx < SR_L_LIM
       SR_Signal = 0;   
       SR_State = 2;
    end
elseif  SR_State == 2
    if PWM_TRIG_State == 2 
        %if raising edge Detected
        SR_State = 0;
    end    
end     

if SR_Signal == 1
    PWM_SR = 1;
else
    PWM_SR = 0;    
end    

end

== matlab function CLLLC_Plant_vLoad_V2/SR Control Pri L ==
  settings: updateMethod=DISCRETE
  data: ITx input; PWM_Trig input; PWM_SR output; Step_Rate parameter
function PWM_SR    = SR_Control(ITx, PWM_Trig, Step_Rate)
 %Constant defines
 
persistent SR_Signal
if isempty(SR_Signal) %Init
    SR_Signal = 0;
end

persistent SR_State
if isempty(SR_State) %Init
    SR_State = 0;
end

persistent PWM_TRIG_State
if isempty(PWM_TRIG_State) %Init
    PWM_TRIG_State = 0;
end

persistent SR_Trig_Count
if isempty(SR_Trig_Count) %Init
    SR_Trig_Count = 0;
end

%SR Trigger Limits - High Side
SR_H_LIM = -8.0;
SR_L_LIM = -5.0;    
SR_H_Trig_Delay = 0.120e-6 / Step_Rate;

if PWM_TRIG_State == 0 %Init
    if PWM_Trig == 0
        PWM_TRIG_State = 1;
    end
elseif PWM_TRIG_State == 1 % Low State Waiting for Raising Edge    
    if PWM_Trig == 1
        PWM_TRIG_State = 2;
    end
elseif PWM_TRIG_State == 2 % Raising Edge Detected 
    PWM_TRIG_State = 3;
elseif PWM_TRIG_State == 3 % @ High State - Wait for Low State 
     if PWM_Trig == 0
        PWM_TRIG_State = 1;
    end
end

if SR_State == 0
    if ITx < SR_H_LIM
        SR_Trig_Count = SR_Trig_Count + 1;
        if SR_Trig_Count > SR_H_Trig_Delay
            SR_State = 1;
            SR_Signal = 1;   
            SR_Trig_Count = 0;
        end
    else
        SR_Trig_Count = 0;        
    end
elseif  SR_State == 1
    if ITx > SR_L_LIM
       SR_Signal = 0;   
       SR_State = 2;
    end
elseif  SR_State == 2
    if PWM_TRIG_State == 2 
        %if raising edge Detected
        SR_State = 0;
    end    
end     

if SR_Signal == 1
    PWM_SR = 1;
else
    PWM_SR = 0;    
end    

end
